simulink model "Monitor"  (R2024a)
settings: Solver=FixedStepDiscrete  StartTime=0.0  StopTime=10.0  RelTol=1e-3  EnableMultiTasking=on
values from neighbouring files (symbols this model uses):
  Dem_EventStatusType : value not decoded    [dict.sldd]
libraries: autosarlibdem x4, simulink x2
settings Model: DataDictionary=dict.sldd  Creator=Administrator  LastModifiedBy=Administrator
settings OptimizationCC: DefaultParameterBehavior=Inlined  EnhancedBackFolding=on  PassReuseOutputArgsAs=Individual arguments  ZeroExternalMemoryAtStartup=off  ZeroInternalMemoryAtStartup=off  OptimizeBlockOrder=speed  DifferentSizesBufferReuse=on  OptimizationCustomize=off  EfficientTunableParamExpr=on
settings DebuggingCC: ParameterTunabilityLossMsg=error
settings SFSimCC: MATLABDynamicMemAlloc=off
settings RTWCC: Description=AUTOSAR  SystemTargetFile=autosar.tlc  GenCodeOnly=on  TemplateMakefile=ert_default_tmf  DataTypeReplacement=CDataTypesFixedWidth
settings CodeAppCC: ForceParamTrailComments=on  IgnoreCustomStorageClasses=off  OperatorAnnotations=on  SimulinkDataObjDesc=on  SFDataObjDesc=on  InsertBlockDesc=on
settings STFCustomTargetCC: MultiwordLength=256  ParMdlRefBuildCompliant=on  CompOptLevelCompliant=on  IncludeMdlTerminateFcn=off  CombineOutputUpdateFcns=on  SuppressErrorStatus=on  ERTCustomFileBanners=on  SupportNonFinite=off  SupportComplex=off  SupportContinuousTime=off  SupportNonInlinedSFcns=off  RemoveResetFunc=on  MATLABClassNameForMDSCustomization=Simulink.SoftwareTarget.ERTCustomization  AutosarCompliant=on  GRTInterface=off  LookupTableObjectStructAxisOrder=2,1,3,4,...  LUTObjectStructOrderEvenSpacing=Size,Table,Breakpoints  SystemTargetFile=autosar.tlc
settings ERTTargetCC: TargetLangStandard=C99 (ISO)  ConcurrentExecutionCompliant=off  IncludeMdlTerminateFcn=off  SuppressErrorStatus=on  SupportNonFinite=off  SupportComplex=off  ModelStepFunctionPrototypeControlCompliant=off  CPPClassGenCompliant=off  AutosarCompliant=on  LookupTableObjectStructAxisOrder=2,1,3,4,...  LUTObjectStructOrderEvenSpacing=Size,Table,Breakpoints  InlinedParameterPlacement=NonHierarchical  ERTCustomFileTemplate=example_file_process.tlc  BooleanTrueId=TRUE  BooleanFalseId=FALSE

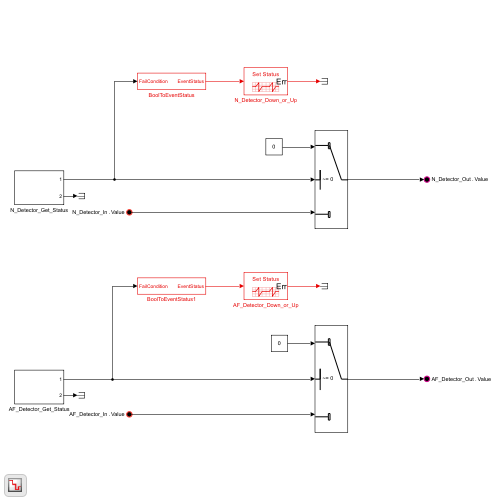
[thumbnail: Simulink's stored preview of the top-level diagram]
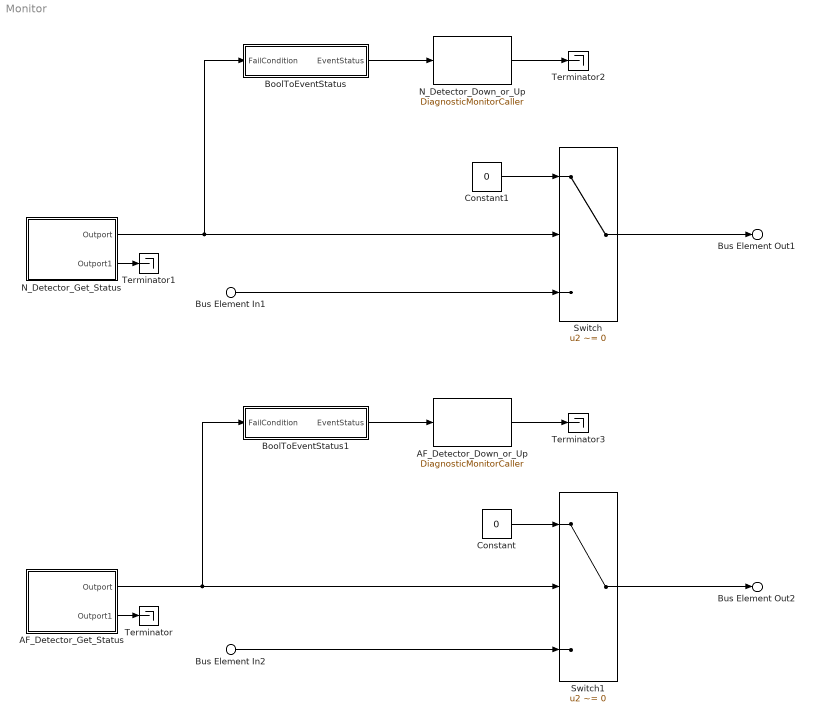
== system Monitor ==
  Bus Element In1 : Inport  PortName=N_Detector_In  Element=Value
  Bus Element In2 : Inport  Port=2  PortName=AF_Detector_In  Element=Value
  AF_Detector_Down_or_Up : autosarlibdem/DiagnosticMonitorCaller  PortName=AutoFogLight_Sensor  Operation=SetEventStatus  Datatype=Enum: Dem_EventStatusType  st=-1  ServiceImpl=autosar.bsw.DemDiagnosticMonitor  SyncToSchema=off
  AF_Detector_Get_Status : Subsystem
  BoolToEventStatus : Subsystem
  BoolToEventStatus1 : Subsystem
  Constant : Constant  Value=0  OutDataTypeStr=single
  Constant1 : Constant  Value=0  OutDataTypeStr=single
  N_Detector_Down_or_Up : autosarlibdem/DiagnosticMonitorCaller  PortName=Night_Sensor  Operation=SetEventStatus  Datatype=Enum: Dem_EventStatusType  st=-1  ServiceImpl=autosar.bsw.DemDiagnosticMonitor  SyncToSchema=off
  N_Detector_Get_Status : Subsystem
  Switch : Switch  Criteria=u2 ~= 0  SaturateOnIntegerOverflow=off  InputSameDT=off
  Switch1 : Switch  Criteria=u2 ~= 0  SaturateOnIntegerOverflow=off  InputSameDT=off
  Terminator{,1..3} (4 alike) : Terminator
  Bus Element Out1 : Outport  Description=|  PortName=N_Detector_Out  Element=Value
      | Sensors detection output values:
      | 0: nothing detected
      | 1: night or fog detected
  Bus Element Out2 : Outport  Description=|  Port=2  PortName=AF_Detector_Out  Element=Value
      | Sensors detection output values:
      | 0: nothing detected
      | 1: night or fog detected
  wires:
  N_Detector_Get_Status/1(Outport) -> BoolToEventStatus/1(FailCondition), Switch/2
  AF_Detector_Get_Status/1(Outport) -> BoolToEventStatus1/1(FailCondition), Switch1/2
  BoolToEventStatus1/1(EventStatus) -> AF_Detector_Down_or_Up/1
  AF_Detector_Down_or_Up/1 -> Terminator3/1
  Constant1/1 -> Switch/1
  Bus Element In2/1 -> Switch1/3
  N_Detector_Down_or_Up/1 -> Terminator2/1
  Constant/1 -> Switch1/1
  Bus Element In1/1 -> Switch/3
  BoolToEventStatus/1(EventStatus) -> N_Detector_Down_or_Up/1
  N_Detector_Get_Status/2(Outport1) -> Terminator1/1
  Switch/1 -> Bus Element Out1/1
  AF_Detector_Get_Status/2(Outport1) -> Terminator/1
  Switch1/1 -> Bus Element Out2/1

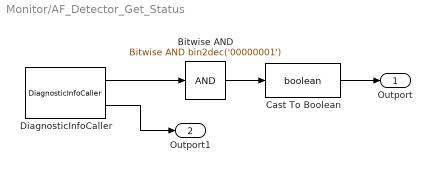
== system Monitor/AF_Detector_Get_Status ==
  Bitwise AND : simulink/Logic and Bit Operations/Bitwise Operator  logicop=AND  UseBitMask=on  BitMask=bin2dec('00000001')  BitMaskRealWorld=Stored Integer
      settings: LibrarySourceBlock=|
      | simulink/Quick Insert/Logic and Bit
      | Operations/Bitwise AND
  Cast To Boolean : DataTypeConversion  OutDataTypeStr=boolean  SaturateOnIntegerOverflow=off  RndMeth=Floor
  DiagnosticInfoCaller : autosarlibdem/DiagnosticInfoCaller  PortName=AF_Detector  Operation=GetEventStatus  st=-1  ServiceImpl=autosar.bsw.DemDiagnosticInfo  SyncToSchema=off
  Outport : Outport
  Outport1 : Outport  Port=2
  wires:
  Bitwise AND/1 -> Cast To Boolean/1
  Cast To Boolean/1 -> Outport/1
  DiagnosticInfoCaller/1 -> Bitwise AND/1
  DiagnosticInfoCaller/2 -> Outport1/1

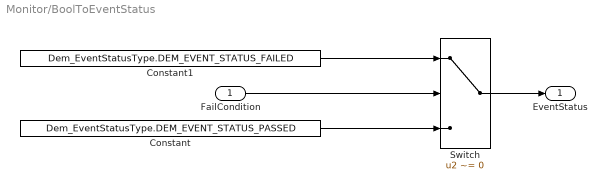
== system Monitor/BoolToEventStatus ==
  FailCondition : Inport
  Constant : Constant  Value=Dem_EventStatusType.DEM_EVENT_STATUS_PASSED
  Constant1 : Constant  Value=Dem_EventStatusType.DEM_EVENT_STATUS_FAILED
  Switch : Switch  Criteria=u2 ~= 0  SaturateOnIntegerOverflow=off  InputSameDT=off
  EventStatus : Outport  VectorParamsAs1DForOutWhenUnconnected=off
  wires:
  FailCondition/1 -> Switch/2
  Constant/1 -> Switch/3
  Constant1/1 -> Switch/1
  Switch/1 -> EventStatus/1

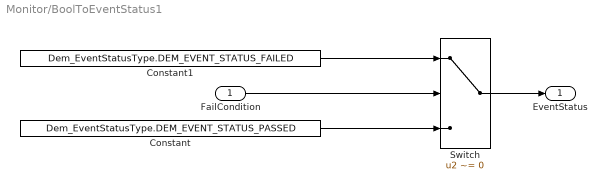
== system Monitor/BoolToEventStatus1 ==
  FailCondition : Inport
  Constant : Constant  Value=Dem_EventStatusType.DEM_EVENT_STATUS_PASSED
  Constant1 : Constant  Value=Dem_EventStatusType.DEM_EVENT_STATUS_FAILED
  Switch : Switch  Criteria=u2 ~= 0  SaturateOnIntegerOverflow=off  InputSameDT=off
  EventStatus : Outport  VectorParamsAs1DForOutWhenUnconnected=off
  wires:
  FailCondition/1 -> Switch/2
  Constant/1 -> Switch/3
  Constant1/1 -> Switch/1
  Switch/1 -> EventStatus/1

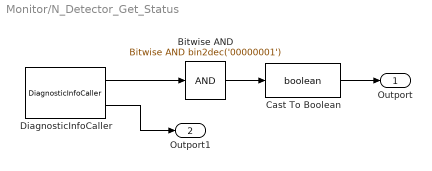
== system Monitor/N_Detector_Get_Status ==
  Bitwise AND : simulink/Logic and Bit Operations/Bitwise Operator  logicop=AND  UseBitMask=on  BitMask=bin2dec('00000001')  BitMaskRealWorld=Stored Integer
      settings: LibrarySourceBlock=|
      | simulink/Quick Insert/Logic and Bit
      | Operations/Bitwise AND
  Cast To Boolean : DataTypeConversion  OutDataTypeStr=boolean  SaturateOnIntegerOverflow=off  RndMeth=Floor
  DiagnosticInfoCaller : autosarlibdem/DiagnosticInfoCaller  PortName=N_Detector  Operation=GetEventStatus  st=-1  ServiceImpl=autosar.bsw.DemDiagnosticInfo  SyncToSchema=off
  Outport : Outport
  Outport1 : Outport  Port=2
  wires:
  Bitwise AND/1 -> Cast To Boolean/1
  Cast To Boolean/1 -> Outport/1
  DiagnosticInfoCaller/1 -> Bitwise AND/1
  DiagnosticInfoCaller/2 -> Outport1/1
